simulink model "sim_cart"  (R2019a)
settings: Solver=VariableStepAuto  StartTime=0.0  StopTime=inf  RelTol=1e-3
libraries: cstblocks x2
settings Model: Creator=mm  LastModifiedBy=Ohnishi

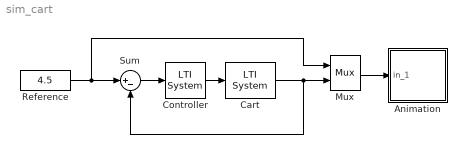
== system sim_cart ==
  Animation : Subsystem  mask(Pendulum plot){RefBlock=Reference}
      mask prompts: RefBlock "DC reference signal block name:"
      mask help: Pendulum plot
      mask Help: Pendulum animation function using Handle graphics.
      mask Display: plot([-5 -5 5 5],[0 3 3 0],[-2 -2 2 2],[0 1 1 0]);
  Cart : cstblocks/LTI System  sys=P  IC=[]
  Controller : cstblocks/LTI System  sys=C  IC=[]
  Mux : Mux  Inputs=2
  Reference : Constant  Value=4.5
  Sum : Sum  Inputs=|+-
  wires:
  Mux/1 -> Animation/1(in_1)
  Sum/1 -> Controller/1
  Reference/1 -> Mux/1, Sum/1
  Controller/1 -> Cart/1
  Cart/1 -> Sum/2, Mux/2

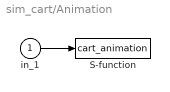
== system sim_cart/Animation ==
  in_1 : Inport
  S-function : S-Function  FunctionName=cart_animation  Parameters=RefBlock  SFunctionDeploymentMode=off  EnableBusSupport=off
      settings: DeleteFcn=pendan([],[],[],'DeleteBlock');
  wires:
  in_1/1 -> S-function/1
